simulink model "lab4_block"  (R2017b)
settings: Solver=VariableStepAuto  StartTime=0.0  StopTime=1.2  RelTol=1e-3
values from neighbouring files (symbols this model uses):
  g1 = G(1), g2=G(2)    [lab4_1.m]
  K = [k11 0; 0 k22]    [harakt.m]    (also in lab4_1.m = -Kisn)
undefined symbols (not defined in the file or in its folder): g2
settings Model: Creator=anton  LastModifiedBy=HONOR

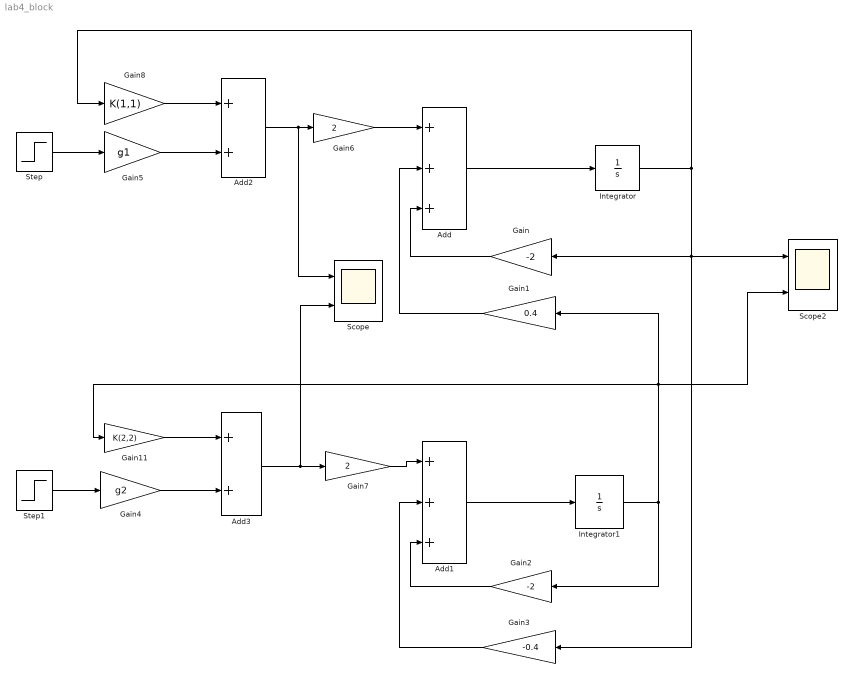
== system lab4_block ==
  Add : Sum  Inputs=+++
  Add1 : Sum  Inputs=+++
  Add2 : Sum
  Add3 : Sum
  Gain : Gain  Gain=-2
  Gain1 : Gain  Gain=0.4
  Gain11 : Gain  Gain=K(2,2)
  Gain2 : Gain  Gain=-2
  Gain3 : Gain  Gain=-0.4
  Gain4 : Gain  Gain=g2
  Gain5 : Gain  Gain=g1
  Gain6 : Gain  Gain=2
  Gain7 : Gain  Gain=2
  Gain8 : Gain  Gain=K(1,1)
  Integrator : Integrator
  Integrator1 : Integrator
  Scope : Scope  NumInputPorts=2
  Scope2 : Scope  NumInputPorts=2
  Step : Step  Time=0  After=1.9  SampleTime=0
  Step1 : Step  Time=0  After=1.9  SampleTime=0
  wires:
  Add/1 -> Integrator/1
  Integrator/1 -> Gain8/1, Gain3/1, Scope2/1, Gain/1
  Gain/1 -> Add/3
  Gain1/1 -> Add/2
  Gain2/1 -> Add1/3
  Gain3/1 -> Add1/2
  Add1/1 -> Integrator1/1
  Step1/1 -> Gain4/1
  Step/1 -> Gain5/1
  Gain4/1 -> Add3/2
  Gain5/1 -> Add2/2
  Gain8/1 -> Add2/1
  Gain11/1 -> Add3/1
  Add2/1 -> Scope/1, Gain6/1
  Gain6/1 -> Add/1
  Add3/1 -> Scope/2, Gain7/1
  Gain7/1 -> Add1/1
  Integrator1/1 -> Scope2/2, Gain11/1, Gain1/1, Gain2/1
